simulink model "InjVlv"  (R2018a)
settings: configuration reference "cs_ert" (kept outside this file)
settings Model: DataDictionary=InjVlv.sldd  Creator=zhoutinglin  LastModifiedBy=zhoutinglin

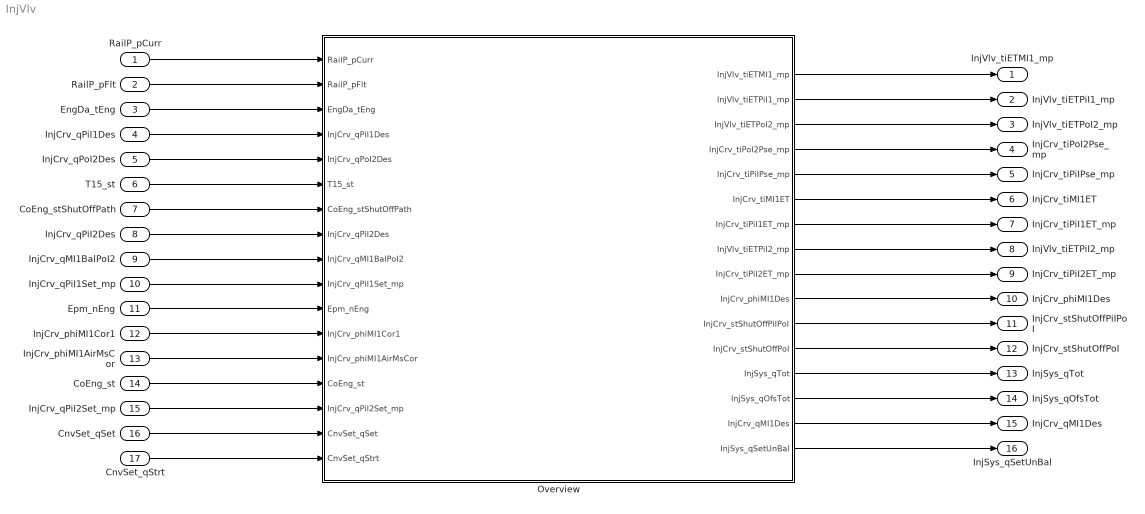
== system InjVlv ==
  RailP_pCurr : Inport
  RailP_pFlt : Inport  Port=2
  EngDa_tEng : Inport  Port=3
  InjCrv_qPiI1Des : Inport  Port=4
  InjCrv_qPoI2Des : Inport  Port=5
  T15_st : Inport  Port=6
  CoEng_stShutOffPath : Inport  Port=7
  InjCrv_qPiI2Des : Inport  Port=8
  InjCrv_qMI1BalPoI2 : Inport  Port=9
  InjCrv_qPiI1Set_mp : Inport  Port=10
  Epm_nEng : Inport  Port=11
  InjCrv_phiMI1Cor1 : Inport  Port=12
  InjCrv_phiMI1AirMsCor : Inport  Port=13
  CoEng_st : Inport  Port=14
  InjCrv_qPiI2Set_mp : Inport  Port=15
  CnvSet_qSet : Inport  Port=16
  CnvSet_qStrt : Inport  Port=17
  Overview : Subsystem
  InjVlv_tiETMI1_mp : Outport
  InjVlv_tiETPiI1_mp : Outport  Port=2
  InjVlv_tiETPoI2_mp : Outport  Port=3
  InjCrv_tiPoI2Pse_mp : Outport  Port=4
  InjCrv_tiPiIPse_mp : Outport  Port=5
  InjCrv_tiMI1ET : Outport  Port=6
  InjCrv_tiPiI1ET_mp : Outport  Port=7
  InjVlv_tiETPiI2_mp : Outport  Port=8
  InjCrv_tiPiI2ET_mp : Outport  Port=9
  InjCrv_phiMI1Des : Outport  Port=10
  InjCrv_stShutOffPiIPoI : Outport  Port=11
  InjCrv_stShutOffPoI : Outport  Port=12
  InjSys_qTot : Outport  Port=13
  InjSys_qOfsTot : Outport  Port=14
  InjCrv_qMI1Des : Outport  Port=15
  InjSys_qSetUnBal : Outport  Port=16
  wires:
  RailP_pCurr/1 -> Overview/1(RailP_pCurr)
  RailP_pFlt/1 -> Overview/2(RailP_pFlt)
  EngDa_tEng/1 -> Overview/3(EngDa_tEng)
  InjCrv_qPiI1Des/1 -> Overview/4(InjCrv_qPiI1Des)
  InjCrv_qPoI2Des/1 -> Overview/5(InjCrv_qPoI2Des)
  T15_st/1 -> Overview/6(T15_st)
  CoEng_stShutOffPath/1 -> Overview/7(CoEng_stShutOffPath)
  InjCrv_qPiI2Des/1 -> Overview/8(InjCrv_qPiI2Des)
  InjCrv_qMI1BalPoI2/1 -> Overview/9(InjCrv_qMI1BalPoI2)
  InjCrv_qPiI1Set_mp/1 -> Overview/10(InjCrv_qPiI1Set_mp)
  Epm_nEng/1 -> Overview/11(Epm_nEng)
  InjCrv_phiMI1Cor1/1 -> Overview/12(InjCrv_phiMI1Cor1)
  InjCrv_phiMI1AirMsCor/1 -> Overview/13(InjCrv_phiMI1AirMsCor)
  CoEng_st/1 -> Overview/14(CoEng_st)
  InjCrv_qPiI2Set_mp/1 -> Overview/15(InjCrv_qPiI2Set_mp)
  CnvSet_qSet/1 -> Overview/16(CnvSet_qSet)
  CnvSet_qStrt/1 -> Overview/17(CnvSet_qStrt)
  Overview/1(InjVlv_tiETMI1_mp) -> InjVlv_tiETMI1_mp/1
  Overview/2(InjVlv_tiETPiI1_mp) -> InjVlv_tiETPiI1_mp/1
  Overview/3(InjVlv_tiETPoI2_mp) -> InjVlv_tiETPoI2_mp/1
  Overview/4(InjCrv_tiPoI2Pse_mp) -> InjCrv_tiPoI2Pse_mp/1
  Overview/5(InjCrv_tiPiIPse_mp) -> InjCrv_tiPiIPse_mp/1
  Overview/6(InjCrv_tiMI1ET) -> InjCrv_tiMI1ET/1
  Overview/7(InjCrv_tiPiI1ET_mp) -> InjCrv_tiPiI1ET_mp/1
  Overview/8(InjVlv_tiETPiI2_mp) -> InjVlv_tiETPiI2_mp/1
  Overview/9(InjCrv_tiPiI2ET_mp) -> InjCrv_tiPiI2ET_mp/1
  Overview/10(InjCrv_phiMI1Des) -> InjCrv_phiMI1Des/1
  Overview/11(InjCrv_stShutOffPiIPoI) -> InjCrv_stShutOffPiIPoI/1
  Overview/12(InjCrv_stShutOffPoI) -> InjCrv_stShutOffPoI/1
  Overview/13(InjSys_qTot) -> InjSys_qTot/1
  Overview/14(InjSys_qOfsTot) -> InjSys_qOfsTot/1
  Overview/15(InjCrv_qMI1Des) -> InjCrv_qMI1Des/1
  Overview/16(InjSys_qSetUnBal) -> InjSys_qSetUnBal/1

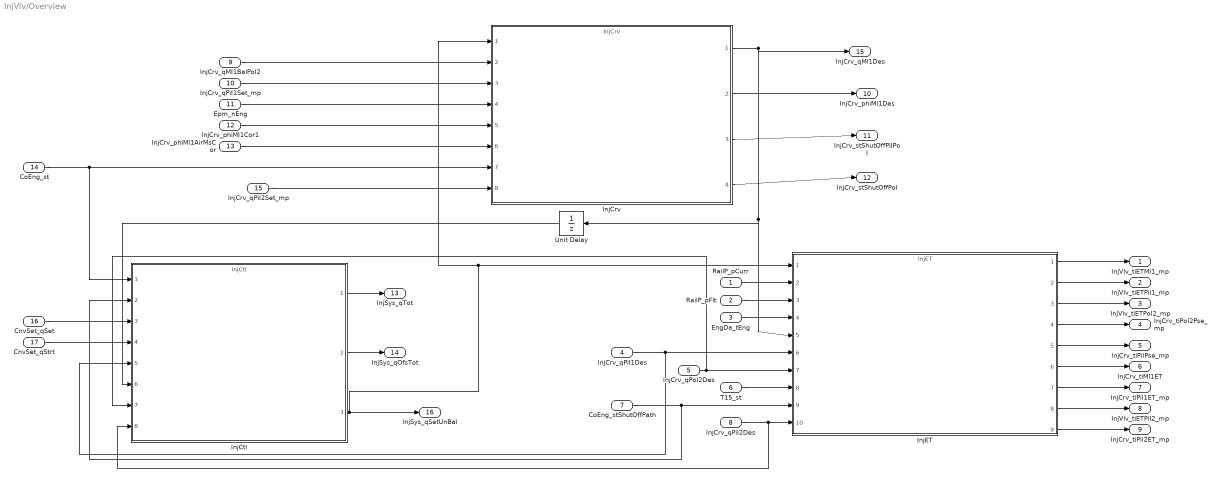
== system InjVlv/Overview ==
  RailP_pCurr : Inport
  RailP_pFlt : Inport  Port=2
  EngDa_tEng : Inport  Port=3
  InjCrv_qPiI1Des : Inport  Port=4
  InjCrv_qPoI2Des : Inport  Port=5
  T15_st : Inport  Port=6
  CoEng_stShutOffPath : Inport  Port=7
  InjCrv_qPiI2Des : Inport  Port=8
  InjCrv_qMI1BalPoI2 : Inport  Port=9
  InjCrv_qPiI1Set_mp : Inport  Port=10
  Epm_nEng : Inport  Port=11
  InjCrv_phiMI1Cor1 : Inport  Port=12
  InjCrv_phiMI1AirMsCor : Inport  Port=13
  CoEng_st : Inport  Port=14
  InjCrv_qPiI2Set_mp : Inport  Port=15
  CnvSet_qSet : Inport  Port=16
  CnvSet_qStrt : Inport  Port=17
  InjCrv : ModelReference  ModelNameDialog=InjCrv  SimulationMode=Normal  ModelReferenceVersion=1.2
  InjCtl : ModelReference  ModelNameDialog=InjCtl  SimulationMode=Normal  ModelReferenceVersion=1.6
  InjET : ModelReference  ModelNameDialog=InjET  SimulationMode=Normal  ModelReferenceVersion=1.3
  Unit Delay : UnitDelay  SampleTime=-1
  InjVlv_tiETMI1_mp : Outport
  InjVlv_tiETPiI1_mp : Outport  Port=2
  InjVlv_tiETPoI2_mp : Outport  Port=3
  InjCrv_tiPoI2Pse_mp : Outport  Port=4
  InjCrv_tiPiIPse_mp : Outport  Port=5
  InjCrv_tiMI1ET : Outport  Port=6
  InjCrv_tiPiI1ET_mp : Outport  Port=7
  InjVlv_tiETPiI2_mp : Outport  Port=8
  InjCrv_tiPiI2ET_mp : Outport  Port=9
  InjCrv_phiMI1Des : Outport  Port=10
  InjCrv_stShutOffPiIPoI : Outport  Port=11
  InjCrv_stShutOffPoI : Outport  Port=12
  InjSys_qTot : Outport  Port=13
  InjSys_qOfsTot : Outport  Port=14
  InjCrv_qMI1Des : Outport  Port=15
  InjSys_qSetUnBal : Outport  Port=16
  wires:
  InjCtl/3 -> InjCrv/1, InjET/1, InjSys_qSetUnBal/1
  InjCrv/1 -> InjET/5, Unit Delay/1, InjCrv_qMI1Des/1
  RailP_pCurr/1 -> InjET/2
  RailP_pFlt/1 -> InjET/3
  EngDa_tEng/1 -> InjET/4
  InjCrv_qPiI1Des/1 -> InjCtl/5, InjET/6
  InjCrv_qPoI2Des/1 -> InjET/7, InjCtl/7
  T15_st/1 -> InjET/8
  CoEng_stShutOffPath/1 -> InjCtl/2, InjET/9
  InjCrv_qPiI2Des/1 -> InjCtl/8, InjET/10
  InjET/1 -> InjVlv_tiETMI1_mp/1
  InjET/2 -> InjVlv_tiETPiI1_mp/1
  InjET/3 -> InjVlv_tiETPoI2_mp/1
  InjET/4 -> InjCrv_tiPoI2Pse_mp/1
  InjET/5 -> InjCrv_tiPiIPse_mp/1
  InjET/6 -> InjCrv_tiMI1ET/1
  InjET/7 -> InjCrv_tiPiI1ET_mp/1
  InjET/8 -> InjVlv_tiETPiI2_mp/1
  InjET/9 -> InjCrv_tiPiI2ET_mp/1
  InjCrv_qMI1BalPoI2/1 -> InjCrv/2
  InjCrv_qPiI1Set_mp/1 -> InjCrv/3
  Epm_nEng/1 -> InjCrv/4
  InjCrv_phiMI1Cor1/1 -> InjCrv/5
  InjCrv_phiMI1AirMsCor/1 -> InjCrv/6
  CoEng_st/1 -> InjCtl/1, InjCrv/7
  InjCrv_qPiI2Set_mp/1 -> InjCrv/8
  InjCrv/2 -> InjCrv_phiMI1Des/1
  InjCrv/3 -> InjCrv_stShutOffPiIPoI/1
  InjCrv/4 -> InjCrv_stShutOffPoI/1
  CnvSet_qSet/1 -> InjCtl/3
  CnvSet_qStrt/1 -> InjCtl/4
  InjCtl/1 -> InjSys_qTot/1
  InjCtl/2 -> InjSys_qOfsTot/1
  Unit Delay/1 -> InjCtl/6
